simulink model "sfcndemo_stvmgain"  (Simulink 6.0)
settings: Solver=FixedStepDiscrete  SolverMode=SingleTasking  StartTime=0.0  StopTime=4.0  FixedStep=.01  RelTol=1e-3
settings Model: Creator=The MathWorks Inc.  LastModifiedBy=batserve  ExtModeTrigMode=oneshot  ExtModeArmWhenConnect=off  ExtModeAutoUpdateStatusClock=off
settings DataIOCC: LimitDataPoints=off  SaveState=on
settings OptimizationCC: BooleanDataType=off
settings DebuggingCC: CheckExecutionContextPreStartOutputMsg=on  CheckExecutionContextRuntimeOutputMsg=on  SolverPrmCheckMsg=none
settings HardwareCC: TargetUnknown=on

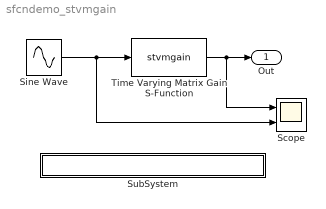
== system sfcndemo_stvmgain ==
  Scope : Scope  NumInputPorts=2
      settings: TimeRange=4  YMin=0~-10  YMax=200~10
  Sine Wave : Sin  Amplitude=[1:10 ]  SampleTime=0
  SubSystem : Subsystem  PropExecContextAcrossSSBoundary=on
      settings: OpenFcn=edit(fullfile(matlabroot,'simulink','src','stvmgain.c'))
      mask Display: disp('matlabroot\simulink\src\stvmgain.c');
  Time Varying Matrix Gain S-Function : S-Function  FunctionName=stvmgain  Parameters=vec, ts  mask(S-function: stvmgain){vec=[1.0 1.25 1.5 1.75 2.0], ts=0.1}
      mask prompts: vec "Input vector:"; ts "Sample Time:"
      mask help: This is a S-function block which calculates time- varying matrix gain function.
  Out : Outport  InitialOutput=0
  wires:
  Time Varying Matrix Gain S-Function/1 -> Out/1, Scope/1
  Sine Wave/1 -> Time Varying Matrix Gain S-Function/1, Scope/2

== system sfcndemo_stvmgain/SubSystem ==
